simulink model "simulation_DIMFCBF"  (R2022a)
settings: Solver=VariableStepAuto  StartTime=0.0  StopTime=simTime  FixedStep=0.01  RelTol=1e-3
values from neighbouring files (symbols this model uses):
  disturbance = true    [setup_DIMFCBF.m]
  gamma = norm_d_inf/(2*k1*alpha)    [setup_DIMFCBF.m]
  Kd = 1    [setup.m]    (also in setup_DIMFCBF.m)
  Kp = 0.2    [setup.m]    (also in setup_DIMFCBF.m)
  M = 10*eye(2)    [setup.m]    (also in setup_DIMFCBF.m = 1*eye(2))
  obstacles = setup_environment(MAP)    [setup_DIMFCBF.m]
  qdotstart = [0,0]    [setup.m]    (also in setup_DIMFCBF.m = [0 ; 0])
  qg = [4, -1]    [setup.m]    (also in setup_DIMFCBF.m = [5, -1])
  qstart = [0,0]    [setup.m]    (also in setup_DIMFCBF.m = [-1 ; 0])
  threshold_skip = 0.0    (= 0)    [setup.m]    (also in setup_DIMFCBF.m)
libraries: slctrlblks x1
settings Model: Creator=mirkomizzoni  LastModifiedBy=dennis

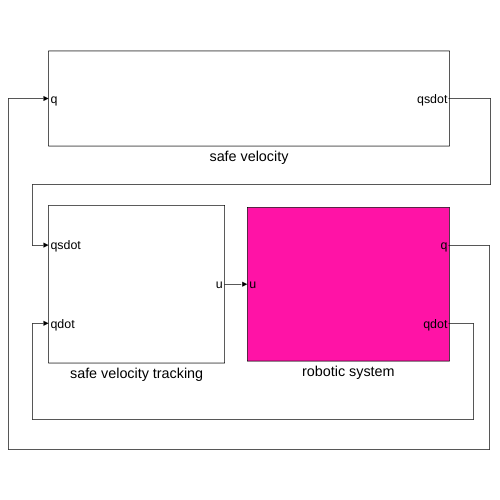
[thumbnail: Simulink's stored preview of the top-level diagram]
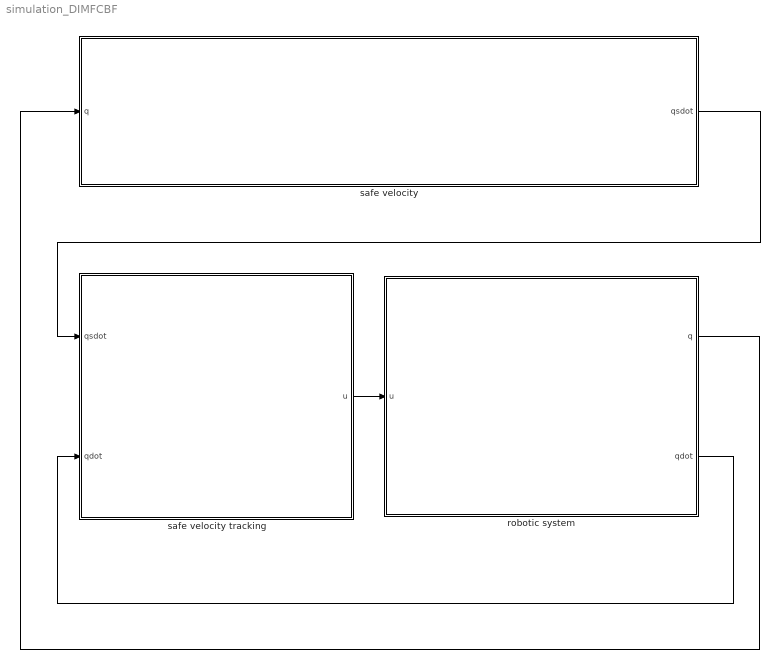
== system simulation_DIMFCBF ==
  robotic system : Subsystem
  safe velocity : Subsystem
  safe velocity tracking : Subsystem
  wires:
  safe velocity tracking/1(u) -> robotic system/1(u)
  safe velocity/1(qsdot) -> safe velocity tracking/1(qsdot)
  robotic system/1(q) -> safe velocity/1(q)
  robotic system/2(qdot) -> safe velocity tracking/2(qdot)

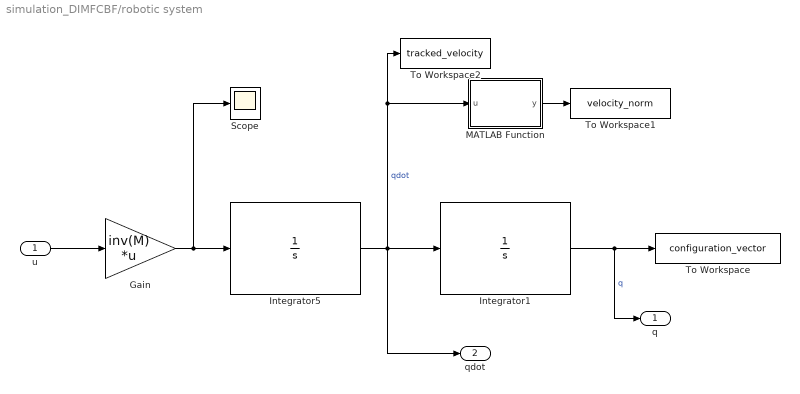
== system simulation_DIMFCBF/robotic system ==
  u : Inport
  Gain : Gain  Gain=inv(M)  Multiplication=Matrix(K*u)
  Integrator1 : Integrator  InitialCondition=qstart
  Integrator5 : Integrator  InitialCondition=qdotstart
  MATLAB Function : MATLAB Function  TreatAsAtomicUnit=on
  Scope : Scope
  To Workspace : ToWorkspace  VariableName=configuration_vector  SaveFormat=Timeseries  SampleTime=0.01
  To Workspace1 : ToWorkspace  VariableName=velocity_norm  SaveFormat=Timeseries  SampleTime=0.01
  To Workspace2 : ToWorkspace  VariableName=tracked_velocity  SaveFormat=Timeseries  SampleTime=0.01
  q : Outport
  qdot : Outport  Port=2
  wires:
  Integrator5/1 -> qdot/1, To Workspace2/1, MATLAB Function/1(u), Integrator1/1  "qdot"
  Integrator1/1 -> q/1, To Workspace/1  "q"
  MATLAB Function/1(y) -> To Workspace1/1
  Gain/1 -> Scope/1, Integrator5/1
  u/1 -> Gain/1

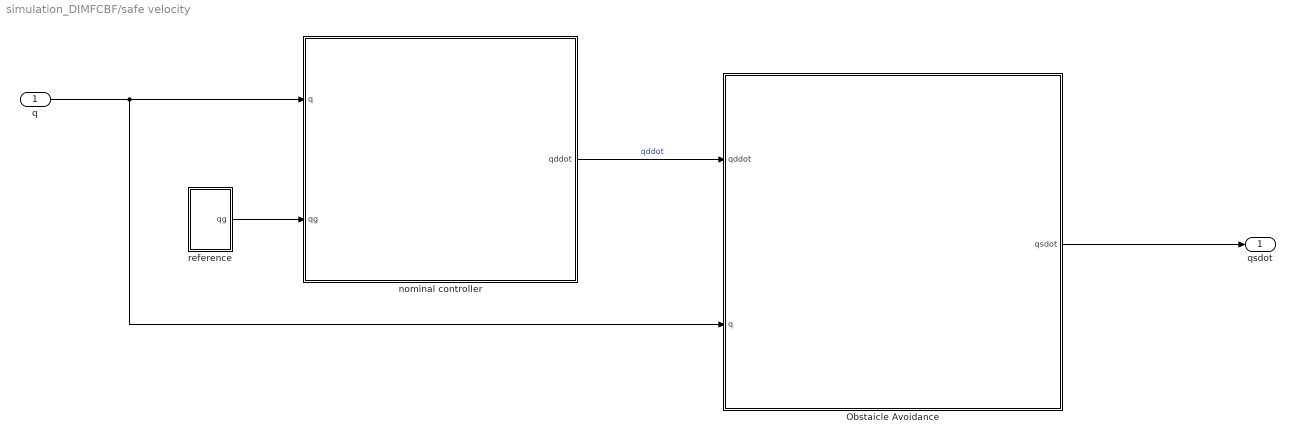
== system simulation_DIMFCBF/safe velocity ==
  q : Inport
  Obstaicle Avoidance : Subsystem
  nominal controller : Subsystem
  reference : Subsystem
  qsdot : Outport
  wires:
  reference/1(qg) -> nominal controller/2(qg)
  nominal controller/1(qddot) -> Obstaicle Avoidance/1(qddot)  "qddot"
  Obstaicle Avoidance/1(qsdot) -> qsdot/1
  q/1 -> nominal controller/1(q), Obstaicle Avoidance/2(q)

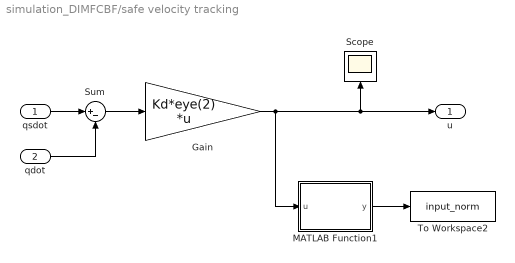
== system simulation_DIMFCBF/safe velocity tracking ==
  qsdot : Inport
  qdot : Inport  Port=2
  Gain : Gain  Gain=Kd*eye(2)  Multiplication=Matrix(K*u)
  MATLAB Function1 : MATLAB Function  TreatAsAtomicUnit=on
  Scope : Scope
  Sum : Sum  Inputs=|+-
  To Workspace2 : ToWorkspace  VariableName=input_norm  SaveFormat=Timeseries  SampleTime=0.01
  u : Outport
  wires:
  qdot/1 -> Sum/2
  Sum/1 -> Gain/1
  MATLAB Function1/1(y) -> To Workspace2/1
  qsdot/1 -> Sum/1
  Gain/1 -> Scope/1, u/1, MATLAB Function1/1(u)

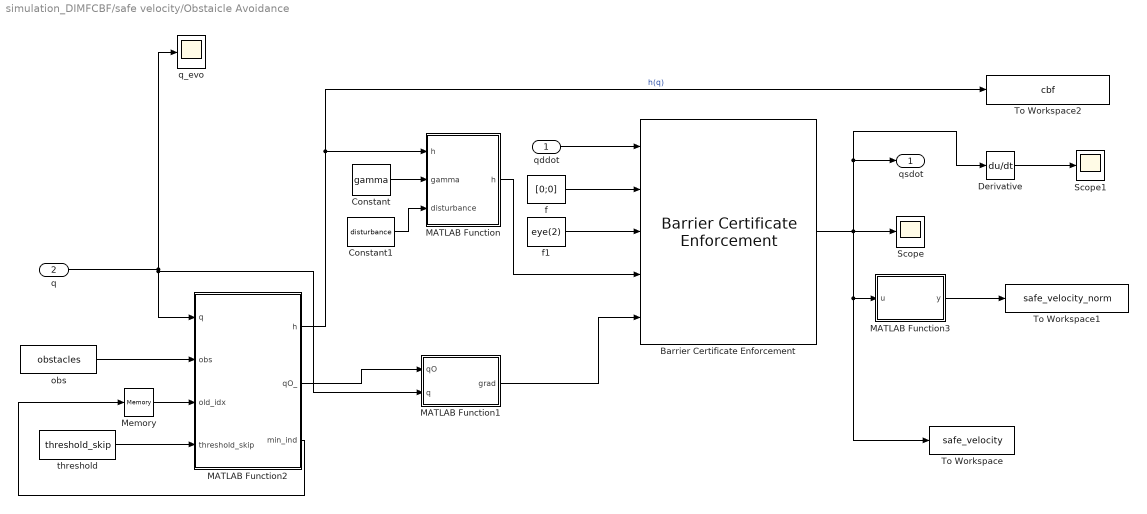
== system simulation_DIMFCBF/safe velocity/Obstaicle Avoidance ==
  qddot : Inport
  q : Inport  Port=2
  Barrier Certificate Enforcement : slctrlblks/Barrier Certificate Enforcement  nx=2  nu=2  nc=1  gamma=alpha  beta=1  external_umax=off  external_umin=off  Ts=0.01  maxiter=200  tol=1e-06  output_exitflag=off
      settings: SourceProductBaseCode=SD
  Constant : Constant  Value=gamma
  Constant1 : Constant  Value=disturbance
  Derivative : Derivative
  MATLAB Function : MATLAB Function  TreatAsAtomicUnit=on
  MATLAB Function1 : MATLAB Function  TreatAsAtomicUnit=on
  MATLAB Function2 : MATLAB Function  TreatAsAtomicUnit=on
  MATLAB Function3 : MATLAB Function  TreatAsAtomicUnit=on
  Memory : Memory  InitialCondition=1
  Scope : Scope
  Scope1 : Scope
  To Workspace : ToWorkspace  VariableName=safe_velocity  SaveFormat=Timeseries  SampleTime=0.01
  To Workspace1 : ToWorkspace  VariableName=safe_velocity_norm  SaveFormat=Timeseries  SampleTime=0.01
  To Workspace2 : ToWorkspace  VariableName=cbf  SaveFormat=Timeseries  SampleTime=0.01
  f : Constant  Value=[0;0]  VectorParams1D=off
  f1 : Constant  Value=eye(2)  VectorParams1D=off
  obs : Constant  Value=obstacles  VectorParams1D=off
  q_evo : Scope
  threshold : Constant  Value=threshold_skip  VectorParams1D=off
  qsdot : Outport
  wires:
  MATLAB Function2/2(qO_) -> MATLAB Function1/1(qO)
  q/1 -> MATLAB Function2/1(q), MATLAB Function1/2(q), q_evo/1
  MATLAB Function2/3(min_ind) -> Memory/1
  MATLAB Function3/1(y) -> To Workspace1/1
  threshold/1 -> MATLAB Function2/4(threshold_skip)
  f/1 -> Barrier Certificate Enforcement/2
  qddot/1 -> Barrier Certificate Enforcement/1
  obs/1 -> MATLAB Function2/2(obs)
  f1/1 -> Barrier Certificate Enforcement/3
  Memory/1 -> MATLAB Function2/3(old_idx)
  Barrier Certificate Enforcement/1 -> To Workspace/1, MATLAB Function3/1(u), Scope/1, Derivative/1, qsdot/1
  MATLAB Function1/1(grad) -> Barrier Certificate Enforcement/5
  MATLAB Function2/1(h) -> To Workspace2/1, MATLAB Function/1("h ")  "h(q)"
  MATLAB Function/1(h) -> Barrier Certificate Enforcement/4
  Constant/1 -> MATLAB Function/2(gamma)
  Derivative/1 -> Scope1/1
  Constant1/1 -> MATLAB Function/3(disturbance)

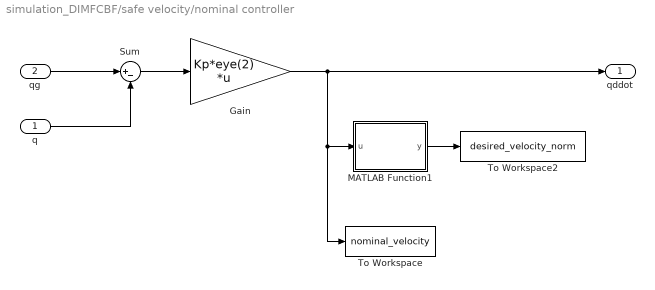
== system simulation_DIMFCBF/safe velocity/nominal controller ==
  q : Inport
  qg : Inport  Port=2
  Gain : Gain  Gain=Kp*eye(2)  Multiplication=Matrix(K*u)
  MATLAB Function1 : MATLAB Function  TreatAsAtomicUnit=on
  Sum : Sum  Inputs=|+-
  To Workspace : ToWorkspace  VariableName=nominal_velocity  SaveFormat=Timeseries  SampleTime=0.01
  To Workspace2 : ToWorkspace  VariableName=desired_velocity_norm  SaveFormat=Timeseries  SampleTime=0.01
  qddot : Outport
  wires:
  MATLAB Function1/1(y) -> To Workspace2/1
  q/1 -> Sum/2
  qg/1 -> Sum/1
  Sum/1 -> Gain/1
  Gain/1 -> To Workspace/1, MATLAB Function1/1(u), qddot/1

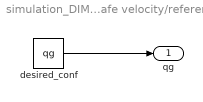
== system simulation_DIMFCBF/safe velocity/reference ==
  desired_conf : Constant  Value=qg
  qg : Outport
  wires:
  desired_conf/1 -> qg/1

== matlab function simulation_DIMFCBF/safe velocity/Obstaicle Avoidance/MATLAB Function1 ==
  data: qO input; grad output; q input
function grad = gradient(qO,q)
   grad = (q-qO)'/norm(q-qO);
end

== matlab function simulation_DIMFCBF/safe velocity/Obstaicle Avoidance/MATLAB Function ==
  data: h input; h output; gamma input; disturbance input
function h = fcn(h, gamma, disturbance)
    if disturbance
        h = h-gamma;
    end
end

== matlab function simulation_DIMFCBF/safe velocity/Obstaicle Avoidance/MATLAB Function2 ==
  data: h output; q input; obs input; qO_ output; min_ind output; old_idx input; threshold_skip input
function [h,qO_,min_ind] = min_dist(q, obs, old_idx, threshold_skip)
% this function is helpful for the computation of the nearest obstacle
% it also returns h' which is the distance between the robot and the
% obstacle taking into account the clearance (for DI)
[~,n] = size(obs);
 o1 = obs(:,1);
 h = norm_obs(q,o1);
 min_ind = 1;
 for i=2:n
        oi = obs(:,i);
        t = norm_obs(q,oi);
        if t<h
            min_ind = i;
            h = t;
        end
    end
    oold = obs(:,old_idx);
    old_dist = norm_obs(q,oold);
    if abs(old_dist-h) < threshold_skip
        qO = oold;
        h = old_dist;
        min_ind = old_idx;
    else
        qO = obs(:,min_ind);
    end
    qO_ = qO(1:2);
end

function min = norm_obs(q, obs)
    min = norm(q-obs(1:2))-obs(3)-obs(4);
end

== matlab function simulation_DIMFCBF/robotic system/MATLAB Function ==
  data: u input; y output
function y = norm_func(u)
        
y = norm(u);

== matlab function simulation_DIMFCBF/safe velocity/Obstaicle Avoidance/MATLAB Function3 ==
  data: u input; y output
function y = norm_func(u)
        
y = norm(u);

== matlab function simulation_DIMFCBF/safe velocity tracking/MATLAB Function1 ==
  data: u input; y output
function y = norm_func(u)
        
y = norm(u);

== matlab function simulation_DIMFCBF/safe velocity/nominal controller/MATLAB Function1 ==
  data: u input; y output
function y = norm_func(u)
        
y = norm(u);
